simulink library "MATLAB_Function_lib"  (R2017b)
settings: Solver=VariableStepAuto  StartTime=0.0  StopTime=10.0  RelTol=1e-3
undefined symbols (not defined in the file or in its folder): Newton, Raphson
libraries: simulink x1
(part 3 of 3)

== system MATLAB_Function_lib/Direction Cosine Matrix to Quaternions/Positive Trace/cos(theta)sin(psi) - (sin(phi)sin(theta)cos(psi) - cos(phi)sin(psi)) ==
  DCM : Inport
  Add : Sum  Inputs=|-+
  Demux : Demux  Outputs=2
  Selector : Selector  InputPortWidth=9  IndexOptions=Index vector (dialog)  Indices=[2 4]  OutputSizes=1
  u(4)-u(2) : Outport
  wires:
  Demux/2 -> Add/2
  Demux/1 -> Add/1
  Selector/1 -> Demux/1
  DCM/1 -> Selector/1
  Add/1 -> u(4)-u(2)/1

== system MATLAB_Function_lib/get_delta_omega/For Iterator Subsystem/Compare To Constant ==
  u : Inport
  Compare : RelationalOperator  Operator===  OutDataTypeStr=boolean  RndMeth=Nearest  InputSameDT=on
  Constant : Constant  DisableCoverage=on  Value=const  OutDataTypeStr=Inherit: Inherit via back propagation
  y : Outport
  wires:
  u/1 -> Compare/1
  Constant/1 -> Compare/2
  Compare/1 -> y/1

== system MATLAB_Function_lib/primary_jet_logic/For Iterator Subsystem/Compare To Constant ==
  u : Inport
  Compare : RelationalOperator  Operator===  OutDataTypeStr=boolean  RndMeth=Nearest  InputSameDT=on
  Constant : Constant  DisableCoverage=on  Value=const  OutDataTypeStr=Inherit: Inherit via back propagation
  y : Outport
  wires:
  u/1 -> Compare/1
  Constant/1 -> Compare/2
  Compare/1 -> y/1

== system MATLAB_Function_lib/primary_jet_logic/For Iterator Subsystem/Compare To Constant1 ==
  u : Inport
  Compare : RelationalOperator  Operator===  OutDataTypeStr=boolean  RndMeth=Nearest  InputSameDT=on
  Constant : Constant  DisableCoverage=on  Value=const  OutDataTypeStr=Inherit: Inherit via back propagation
  y : Outport
  wires:
  u/1 -> Compare/1
  Constant/1 -> Compare/2
  Compare/1 -> y/1

== system MATLAB_Function_lib/primary_jet_logic/For Iterator Subsystem/Compare To Constant2 ==
  u : Inport
  Compare : RelationalOperator  Operator===  OutDataTypeStr=boolean  RndMeth=Nearest  InputSameDT=on
  Constant : Constant  DisableCoverage=on  Value=const  OutDataTypeStr=Inherit: Inherit via back propagation
  y : Outport
  wires:
  u/1 -> Compare/1
  Constant/1 -> Compare/2
  Compare/1 -> y/1

== system MATLAB_Function_lib/primary_jet_logic/For Iterator Subsystem/Compare To Constant3 ==
  u : Inport
  Compare : RelationalOperator  Operator=~=  OutDataTypeStr=boolean  RndMeth=Nearest  InputSameDT=on
  Constant : Constant  DisableCoverage=on  Value=const  OutDataTypeStr=Inherit: Inherit via back propagation
  y : Outport
  wires:
  u/1 -> Compare/1
  Constant/1 -> Compare/2
  Compare/1 -> y/1

== system MATLAB_Function_lib/primary_jet_logic/For Iterator Subsystem/Compare To Constant4 ==
  u : Inport
  Compare : RelationalOperator  Operator===  OutDataTypeStr=boolean  RndMeth=Nearest  InputSameDT=on
  Constant : Constant  DisableCoverage=on  Value=const  OutDataTypeStr=Inherit: Inherit via back propagation
  y : Outport
  wires:
  u/1 -> Compare/1
  Constant/1 -> Compare/2
  Compare/1 -> y/1

== system MATLAB_Function_lib/Direction Cosine Matrix to Quaternions/Negative Trace/Maximum Value at DCM(1,1)/cos(phi)sin(theta)cos(psi) + sin(phi)sin(psi) -sin(theta) ==
  DCM : Inport
  Add : Sum  Inputs=++|
  Demux : Demux  Outputs=2
  Selector : Selector  InputPortWidth=9  IndexOptions=Index vector (dialog)  Indices=[3 7]  OutputSizes=1
  u(3)+u(7) : Outport
  wires:
  Selector/1 -> Demux/1
  Demux/1 -> Add/1
  Demux/2 -> Add/2
  Add/1 -> u(3)+u(7)/1
  DCM/1 -> Selector/1

== system MATLAB_Function_lib/Direction Cosine Matrix to Quaternions/Negative Trace/Maximum Value at DCM(1,1)/cos(theta)sin(phi) - (cos(phi)sin(theta)sin(psi) - sin(phi)cos(psi)) ==
  DCM : Inport
  Add : Sum  Inputs=|-+
  Demux : Demux  Outputs=2
  Selector : Selector  InputPortWidth=9  IndexOptions=Index vector (dialog)  Indices=[6 8]  OutputSizes=1
  u(8)-u(6) : Outport
  wires:
  Demux/2 -> Add/2
  Demux/1 -> Add/1
  Selector/1 -> Demux/1
  Add/1 -> u(8)-u(6)/1
  DCM/1 -> Selector/1

== system MATLAB_Function_lib/Direction Cosine Matrix to Quaternions/Negative Trace/Maximum Value at DCM(1,1)/cos(theta)sin(psi) + (sin(phi)sin(theta)cos(psi) - cos(phi)sin(psi)) ==
  DCM : Inport
  Add : Sum  Inputs=|++
  Demux : Demux  Outputs=2
  Selector : Selector  InputPortWidth=9  IndexOptions=Index vector (dialog)  Indices=[2 4]  OutputSizes=1
  u(4)+u(2) : Outport
  wires:
  Demux/2 -> Add/2
  Demux/1 -> Add/1
  Selector/1 -> Demux/1
  DCM/1 -> Selector/1
  Add/1 -> u(4)+u(2)/1

== system MATLAB_Function_lib/Direction Cosine Matrix to Quaternions/Negative Trace/Maximum Value at DCM(1,1)/if s~=0; s=0.5//s ==
  s : Inport
  Constant1 : Constant  Value=0.5  OutDataTypeStr=Inherit: Inherit via back propagation
  Constant2 : Constant  Value=[0 1]  OutDataTypeStr=Inherit: Inherit via back propagation
  Demux : Demux  Outputs=2
  Mux : Mux  Inputs=2
  Product : Product  Inputs=*/  RndMeth=Zero
  Switch : Switch  Criteria=u2 ~= 0  SaturateOnIntegerOverflow=on  InputSameDT=on
  "s " : Outport
  wires:
  Product/1 -> "s "/1
  Constant2/1 -> Switch/3
  Switch/1 -> Demux/1
  s/1 -> Mux/2, Switch/2
  Mux/1 -> Switch/1
  Constant1/1 -> Mux/1
  Demux/2 -> Product/2
  Demux/1 -> Product/1

== system MATLAB_Function_lib/Direction Cosine Matrix to Quaternions/Negative Trace/Maximum Value at DCM(1,1)/u(1) -(u(5)+u(9)) +1 ==
  DCM : Inport
  Add : Sum  Inputs=+--+
  Constant : Constant  OutDataTypeStr=Inherit: Inherit via back propagation
  Demux : Demux  Outputs=3
  Selector : Selector  InputPortWidth=9  IndexOptions=Index vector (dialog)  Indices=[1 5 9]  OutputSizes=1
  out : Outport
  wires:
  Demux/3 -> Add/3
  Demux/1 -> Add/1
  Demux/2 -> Add/2
  Selector/1 -> Demux/1
  Constant/1 -> Add/4
  DCM/1 -> Selector/1
  Add/1 -> out/1

== system MATLAB_Function_lib/Direction Cosine Matrix to Quaternions/Negative Trace/Maximum Value at DCM(2,2)/cos(phi)sin(theta)cos(psi) + sin(phi)sin(psi) +sin(theta) ==
  DCM : Inport
  Add : Sum  Inputs=+-|
  Demux : Demux  Outputs=2
  Selector : Selector  InputPortWidth=9  IndexOptions=Index vector (dialog)  Indices=[3 7]  OutputSizes=1
  u(3)-u(7) : Outport
  wires:
  Selector/1 -> Demux/1
  Demux/1 -> Add/1
  DCM/1 -> Selector/1
  Demux/2 -> Add/2
  Add/1 -> u(3)-u(7)/1

== system MATLAB_Function_lib/Direction Cosine Matrix to Quaternions/Negative Trace/Maximum Value at DCM(2,2)/cos(theta)sin(phi) + (cos(phi)sin(theta)sin(psi) - sin(phi)cos(psi)) ==
  DCM : Inport
  Add : Sum  Inputs=|++
  Demux : Demux  Outputs=2
  Selector : Selector  InputPortWidth=9  IndexOptions=Index vector (dialog)  Indices=[6 8]  OutputSizes=1
  u(8)+u(6) : Outport
  wires:
  Demux/2 -> Add/2
  Demux/1 -> Add/1
  Selector/1 -> Demux/1
  DCM/1 -> Selector/1
  Add/1 -> u(8)+u(6)/1

== system MATLAB_Function_lib/Direction Cosine Matrix to Quaternions/Negative Trace/Maximum Value at DCM(2,2)/cos(theta)sin(psi) + (sin(phi)sin(theta)cos(psi) - cos(phi)sin(psi)) ==
  DCM : Inport
  Add : Sum  Inputs=|++
  Demux : Demux  Outputs=2
  Selector : Selector  InputPortWidth=9  IndexOptions=Index vector (dialog)  Indices=[2 4]  OutputSizes=1
  u(4)+u(2) : Outport
  wires:
  Demux/2 -> Add/2
  Demux/1 -> Add/1
  Selector/1 -> Demux/1
  Add/1 -> u(4)+u(2)/1
  DCM/1 -> Selector/1

== system MATLAB_Function_lib/Direction Cosine Matrix to Quaternions/Negative Trace/Maximum Value at DCM(2,2)/if s~=0; s=0.5//s ==
  s : Inport
  Constant1 : Constant  Value=0.5  OutDataTypeStr=Inherit: Inherit via back propagation
  Constant2 : Constant  Value=[0 1]  OutDataTypeStr=Inherit: Inherit via back propagation
  Demux : Demux  Outputs=2
  Mux : Mux  Inputs=2
  Product : Product  Inputs=*/  RndMeth=Zero
  Switch : Switch  Criteria=u2 ~= 0  SaturateOnIntegerOverflow=on  InputSameDT=on
  "s " : Outport
  wires:
  Demux/1 -> Product/1
  Demux/2 -> Product/2
  Constant1/1 -> Mux/1
  Mux/1 -> Switch/1
  s/1 -> Switch/2, Mux/2
  Switch/1 -> Demux/1
  Constant2/1 -> Switch/3
  Product/1 -> "s "/1

== system MATLAB_Function_lib/Direction Cosine Matrix to Quaternions/Negative Trace/Maximum Value at DCM(2,2)/u(5) -(u(1)+u(9)) +1 ==
  DCM : Inport
  Add : Sum  Inputs=-+-+
  Constant : Constant  OutDataTypeStr=Inherit: Inherit via back propagation
  Demux : Demux  Outputs=3
  Selector : Selector  InputPortWidth=9  IndexOptions=Index vector (dialog)  Indices=[1 5 9]  OutputSizes=1
  out : Outport
  wires:
  Demux/3 -> Add/3
  Demux/1 -> Add/1
  Demux/2 -> Add/2
  Selector/1 -> Demux/1
  Add/1 -> out/1
  DCM/1 -> Selector/1
  Constant/1 -> Add/4

== system MATLAB_Function_lib/Direction Cosine Matrix to Quaternions/Negative Trace/Maximum Value at DCM(3,3)/cos(phi)sin(theta)cos(psi) + sin(phi)sin(psi) -sin(theta) ==
  DCM : Inport
  Add : Sum  Inputs=++|
  Demux : Demux  Outputs=2
  Selector : Selector  InputPortWidth=9  IndexOptions=Index vector (dialog)  Indices=[3 7]  OutputSizes=1
  u(3)+u(7) : Outport
  wires:
  Selector/1 -> Demux/1
  Demux/1 -> Add/1
  Demux/2 -> Add/2
  DCM/1 -> Selector/1
  Add/1 -> u(3)+u(7)/1

== system MATLAB_Function_lib/Direction Cosine Matrix to Quaternions/Negative Trace/Maximum Value at DCM(3,3)/cos(theta)sin(phi) + (cos(phi)sin(theta)sin(psi) - sin(phi)cos(psi)) ==
  DCM : Inport
  Add : Sum  Inputs=|++
  Demux : Demux  Outputs=2
  Selector : Selector  InputPortWidth=9  IndexOptions=Index vector (dialog)  Indices=[6 8]  OutputSizes=1
  u(8)+u(6) : Outport
  wires:
  Demux/2 -> Add/2
  Demux/1 -> Add/1
  Selector/1 -> Demux/1
  Add/1 -> u(8)+u(6)/1
  DCM/1 -> Selector/1

== system MATLAB_Function_lib/Direction Cosine Matrix to Quaternions/Negative Trace/Maximum Value at DCM(3,3)/cos(theta)sin(psi) - (sin(phi)sin(theta)cos(psi) - cos(phi)sin(psi)) ==
  DCM : Inport
  Add : Sum  Inputs=|-+
  Demux : Demux  Outputs=2
  Selector : Selector  InputPortWidth=9  IndexOptions=Index vector (dialog)  Indices=[2 4]  OutputSizes=1
  u(4)-u(2) : Outport
  wires:
  Demux/2 -> Add/2
  Demux/1 -> Add/1
  Selector/1 -> Demux/1
  Add/1 -> u(4)-u(2)/1
  DCM/1 -> Selector/1

== system MATLAB_Function_lib/Direction Cosine Matrix to Quaternions/Negative Trace/Maximum Value at DCM(3,3)/if s~=0; s=0.5//s ==
  s : Inport
  Constant1 : Constant  Value=0.5  OutDataTypeStr=Inherit: Inherit via back propagation
  Constant2 : Constant  Value=[0 1]  OutDataTypeStr=Inherit: Inherit via back propagation
  Demux : Demux  Outputs=2
  Mux : Mux  Inputs=2
  Product : Product  Inputs=*/  RndMeth=Zero
  Switch : Switch  Criteria=u2 ~= 0  SaturateOnIntegerOverflow=on  InputSameDT=on
  "s " : Outport
  wires:
  Product/1 -> "s "/1
  Constant2/1 -> Switch/3
  Switch/1 -> Demux/1
  s/1 -> Mux/2, Switch/2
  Mux/1 -> Switch/1
  Constant1/1 -> Mux/1
  Demux/2 -> Product/2
  Demux/1 -> Product/1

== system MATLAB_Function_lib/Direction Cosine Matrix to Quaternions/Negative Trace/Maximum Value at DCM(3,3)/u(9) -(u(1)+u(5)) +1 ==
  DCM : Inport
  Add : Sum  Inputs=--++
  Constant : Constant  OutDataTypeStr=Inherit: Inherit via back propagation
  Demux : Demux  Outputs=3
  Selector : Selector  InputPortWidth=9  IndexOptions=Index vector (dialog)  Indices=[1 5 9]  OutputSizes=1
  out : Outport
  wires:
  Demux/3 -> Add/3
  Demux/1 -> Add/1
  Demux/2 -> Add/2
  Selector/1 -> Demux/1
  Add/1 -> out/1
  DCM/1 -> Selector/1
  Constant/1 -> Add/4
